simulink model "UDP_send_recieve"  (R2018a)
settings: Solver=FixedStepAuto  StartTime=0.0  StopTime=inf  FixedStep=0.001  MaxStep=0.033333333333333333  RelTol=1e-3
libraries: svdutilitieslib x2, xpcrtudplib x2, aerolibanimutils x1
settings Model: Creator=gyga  LastModifiedBy=gyga

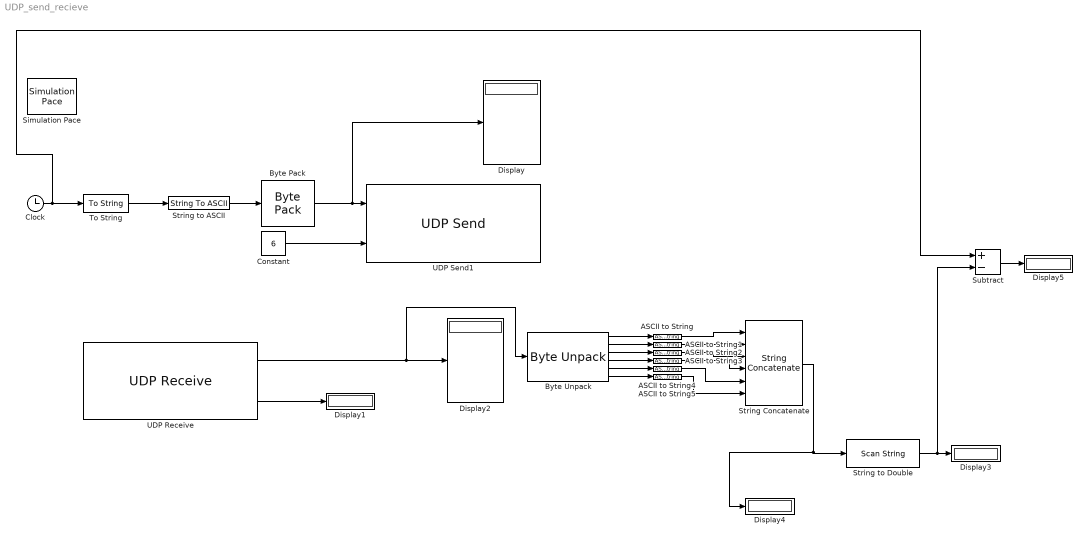
== system UDP_send_recieve ==
  ASCII to String{,1..5} (6 alike) : ASCIIToString
  Byte Pack : svdutilitieslib/Byte Pack  maskPackedDataType=uint8  datatypes={'uint8'}  byteAlign=1  blockPlatform=arduinoert
      settings: SourceProductName=Simulink Support Package for Arduino Hardware  SourceProductBaseCode=ARDUINO
  Byte Unpack : svdutilitieslib/Byte Unpack  dimensions={1, 1, 1, 1, 1, 1}  datatypes={'uint8', 'uint8', 'uint8', 'uint8', 'uint8', 'uint8'}  byteAlign=1  blockPlatform=arduinoert
      settings: SourceProductName=Simulink Support Package for Arduino Hardware  SourceProductBaseCode=ARDUINO
  Clock : Clock
  Constant : Constant  Value=6
  Display{,1..5} (6 alike) : Display
  Simulation Pace : aerolibanimutils/Simulation Pace  SimulationPace=1  SleepMode=MATLAB Thread  OutputPaceError=off  SampleTime=1/100
  String Concatenate : StringConcatenate  Inputs=6
  String to ASCII : StringToASCII  MaximumLength=6
  String to Double : ScanString  Format="\"%lf\""
  Subtract : Sum  Inputs=+-
  To String : ToString
  UDP Receive : xpcrtudplib/UDP Receive  ipAddressVal=Use host-target connection  localPort=25002  rcvWidth=6  rcvFmAny=on  fmAddress=0.0.0.0  rcvMulticast=off  multicastAddress=[]  maxUDPQueue=8  sampleTime=-1
      settings: SourceProductName=Simulink Real-Time
  UDP Send1 : xpcrtudplib/UDP Send  ipAddressVal=Use host-target connection  localPort=25001  toAddress=127.0.0.1  toPort=25003  sampleTime=-1
      settings: SourceProductName=Simulink Real-Time  SourceProductBaseCode=XP
  wires:
  Clock/1 -> Subtract/1, To String/1
  To String/1 -> String to ASCII/1
  String to ASCII/1 -> Byte Pack/1
  Byte Pack/1 -> Display/1, UDP Send1/1
  Constant/1 -> UDP Send1/2
  UDP Receive/1 -> Byte Unpack/1, Display2/1
  UDP Receive/2 -> Display1/1
  Byte Unpack/1 -> ASCII to String/1
  ASCII to String/1 -> String Concatenate/1
  ASCII to String2/1 -> String Concatenate/3
  Byte Unpack/3 -> ASCII to String2/1
  ASCII to String4/1 -> String Concatenate/5
  Byte Unpack/5 -> ASCII to String4/1
  ASCII to String1/1 -> String Concatenate/2
  ASCII to String3/1 -> String Concatenate/4
  ASCII to String5/1 -> String Concatenate/6
  String Concatenate/1 -> String to Double/1, Display4/1
  Byte Unpack/2 -> ASCII to String1/1
  Byte Unpack/4 -> ASCII to String3/1
  Byte Unpack/6 -> ASCII to String5/1
  String to Double/1 -> Subtract/2, Display3/1
  Subtract/1 -> Display5/1
